simulink model "Copy_of_mpcACCWithSensorFusion"  (R2023b)
settings: Solver=FixedStepAuto  StartTime=0.0  StopTime=34  FixedStep=0.1  RelTol=1e-3
values from neighbouring files (symbols this model uses):
  pfcsubsystem_data =     [pfc_controller_data.mat]    (also in pfc_data.mat; pfc_subsystem_data.mat)
  posSelector = [1,0,0,0,0,0; 0,0,1,0,0,0]    [setUpACCWorkspaceVars.m]
  Ts = 0.1    [mainACCcode.m]    (also in setUpACCWorkspaceVars.m)
undefined symbols (not defined in the file or in its folder): hasLag, InitialLongVel, NumEgoStates, PredictionHorizon
libraries: mpcsigdimcheck_private x19, simulink x2, mpclib x2, trackingutilitieslib x1, drivinglib x1
(part 2 of 2)

== matlab function Copy_of_mpcACCWithSensorFusion/MPC Controller /PFC controller/MPC Models/MPC Model with Spacing Control/Adaptive Model with Spacing Control ==
  data: Ts input; A output; Vx input; Ag input; Bg input; Cg input; lag input; B output; C output; D output
function [A,B,C,D] = getAdaptiveMPCModel(Ts,Vx, Ag, Bg, Cg, lag)
% Get discrete state-space model for Adaptive MPC with sample time Ts.
% Called by the 'Path Following Control System' Block.

% Inputs:
%   Ts:               mask variable for sample time
%   Vx:               mask inport for longitudinal velocity
%   Ag,Bg,Cg:         continuous or discrete vehicle model with sample time Ts
% Outputs:
%   A,B,C,D:          discrete time model for adaptive MPC

%   Author: Meng Xia, Rong Chen
%   Copyright 2017-2018 The MathWorks, Inc.

% Discrete MPC model
[A,B,C,D] = pfcblock_utilGetDTModelHasLagForMPCHasSpacingCtrl(Ts,Vx,Ag,Bg,Cg,lag);

== matlab function Copy_of_mpcACCWithSensorFusion/Tracking and Sensor Fusion/Find Lead Car ==
  data: confirmedTracks input; x output size=[1 1]; vx output size=[1 1]; lane input; mioTrackIndex output; positionSelector input
function [x,vx,mioTrackIndex] = findLeadCar(confirmedTracks, lane, positionSelector)
% This function finds the lead car: a car in front of the ego car that
% satisfies all the criteria below:
% * Within the ego car's lane.
% * In front of the ego car.
% * Closest to the ego car.

% Note: If you change state definition, change the following:
%       State = [x;vx;y;vy;z;vz] (3D constant velocity)
numStates = 6;

% Initialize outputs and parameters
maxX = cast(1000, 'like', confirmedTracks.Tracks(1).State);  % Far enough forward so that no track is expected to exceed this distance
mioTrackIndex = 0;

% If lane detection is not available, the ego car is assumed to be located
% in the middle of its lane. The lane width is assumed to be 3.6m, typical
% highway lane width.
laneWidth = 3.6;
halfLaneWidth = laneWidth/2;

if lane.Left.Strength > 0.01
    lb = [lane.Left.CurvatureDerivative/6,...
        lane.Left.Curvature/2,...
        lane.Left.HeadingAngle,...
        lane.Left.LateralOffset];
else
    lb = single([0,0,0,halfLaneWidth]);
end

if lane.Right.Strength > 0.01
    rb = [lane.Right.CurvatureDerivative/6,...
        lane.Right.Curvature/2,...
        lane.Right.HeadingAngle,...
        lane.Right.LateralOffset];
else
    rb = single([0,0,0,-halfLaneWidth]);    
end

for i = 1:confirmedTracks.NumTracks
    position = positionSelector * confirmedTracks.Tracks(i).State;
    x = position(1); % Longitudinal position of the track relative to ego
    y = position(2); % Lateral position of the track relative to ego
    
    if x < maxX && x > 0 % No point checking otherwise

        yleftLane  = polyval(lb,x); % lateral position of left lane
        yrightLane = polyval(rb,x); % lateral position of right lane
        
        % Find a new lead car
        if (yrightLane <= y) && (y <= yleftLane)
            maxX = x;
            mioTrackIndex(:) = i;
        end
    end
end

if mioTrackIndex>0
    mioState = confirmedTracks.Tracks(mioTrackIndex).State;
else
    mioState = inf(numStates,1,'like',confirmedTracks.Tracks(1).State);
end

% Output:
x = mioState(1);    % Longitudinal position of the lead car
vx = mioState(2);   % Longitudinal velocity of the lead car

== matlab function Copy_of_mpcACCWithSensorFusion/MPC Controller /PFC controller/Data Processing for MPC Controller/DataTypeConversion_extmv ==
  data: u input size=[2 1]; y output; isDouble parameter
function y = fcn(u,isDouble)
if isDouble
    if isa(u,'double')
        y = u;
    else
        y = double(u);
    end
else
    if isa(u,'single')
        y = u;
    else
        y = single(u);
    end
end

== matlab function Copy_of_mpcACCWithSensorFusion/Estimate Lane Center/MATLAB Function ==
  data: lanes input
  events: fcnLeftAndRight output FUNCTION_CALL_EVENT; fcnLeftOnly output FUNCTION_CALL_EVENT; fcnRightOnly output FUNCTION_CALL_EVENT; fcnNone output FUNCTION_CALL_EVENT
function fcn(lanes)

leftStrength  = lanes.Left.Strength;
rightStrength = lanes.Right.Strength;

if (leftStrength > 0) && (rightStrength > 0)
   fcnLeftAndRight();
   
elseif leftStrength > 0
    fcnLeftOnly();
    
elseif rightStrength > 0
    fcnRightOnly();
    
else
    fcnNone();
end
